simulink model "untitled"  (R2023b)
settings: Solver=VariableStepAuto  StartTime=0.0  StopTime=10.0  RelTol=1e-3
settings Model: Creator=ousso  LastModifiedBy=ousso

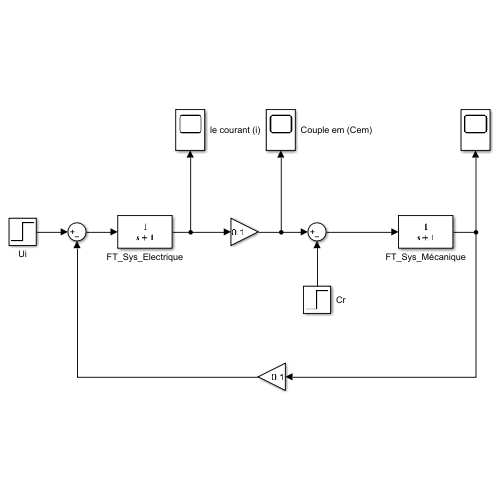
[thumbnail: Simulink's stored preview of the top-level diagram]
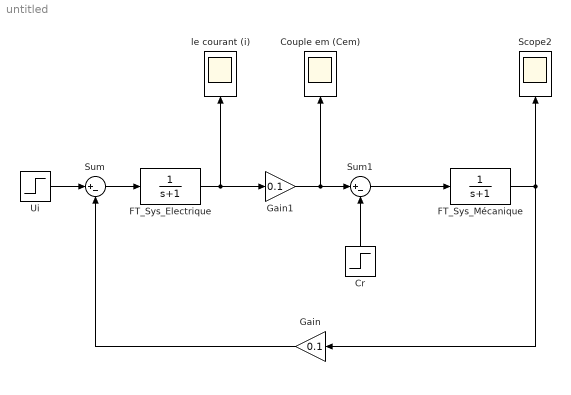
== system untitled ==
  Couple em (Cem) : Scope
  Cr : Step  SampleTime=0
  FT_Sys_Electrique : TransferFcn  Denominator=[1 1]
  FT_Sys_Mécanique : TransferFcn  Denominator=[1 1]
  Gain : Gain  Gain=0.1
  Gain1 : Gain  Gain=0.1
  Scope2 : Scope
  Sum : Sum  Inputs=|+-
  Sum1 : Sum  Inputs=|+-
  Ui : Step  SampleTime=0
  le courant (i) : Scope
  wires:
  FT_Sys_Electrique/1 -> Gain1/1, le courant (i)/1
  Ui/1 -> Sum/1
  Sum/1 -> FT_Sys_Electrique/1
  Gain1/1 -> Sum1/1, Couple em (Cem)/1
  Sum1/1 -> FT_Sys_Mécanique/1
  Gain/1 -> Sum/2
  Cr/1 -> Sum1/2
  FT_Sys_Mécanique/1 -> Gain/1, Scope2/1
